simulink model "pedal"  (R2021a)
settings: Solver=FixedStepDiscrete  StartTime=0.0  StopTime=12  FixedStep=1e-3  RelTol=1e-3  EnableMultiTasking=on
undefined symbols (not defined in the file): APP_Modes, sigbuilder_block
settings Model: SILPILModeSetting=veronly  ExtModeTrigDuration=2  Creator=Beshary  LastModifiedBy=Beshary
settings DataIOCC: ExternalInput=[t, S1,S2]  LoadExternalInput=on  SaveFormat=Array
settings OptimizationCC: EnhancedBackFolding=on  PassReuseOutputArgsAs=Individual arguments  ZeroExternalMemoryAtStartup=off  ZeroInternalMemoryAtStartup=off  MaxStackSize=64  OptimizeBlockOrder=speed  DifferentSizesBufferReuse=on  OptimizationCustomize=off  EfficientTunableParamExpr=on
settings DebuggingCC: ParameterTunabilityLossMsg=error
settings HardwareCC: ProdBitPerInt=16  ProdBitPerPointer=16  ProdBitPerSizeT=16  ProdBitPerPtrDiffT=16  ProdLargestAtomicFloat=None  ProdWordSize=8  ProdHWDeviceType=Atmel->AVR
settings SFSimCC: MATLABDynamicMemAlloc=off
settings RTWCC: SystemTargetFile=ert.tlc  HardwareBoard=Arduino Uno  TemplateMakefile=ert_default_tmf  Toolchain=Arduino AVR  BuildConfiguration=Faster Runs
settings CodeAppCC: ForceParamTrailComments=on  IgnoreCustomStorageClasses=off  OperatorAnnotations=on  SimulinkDataObjDesc=on  SFDataObjDesc=on  InsertBlockDesc=on
settings ERTTargetCC: SupportContinuousTime=on  SupportVariableSizeSignals=on  ExtModeStaticAllocSize=250

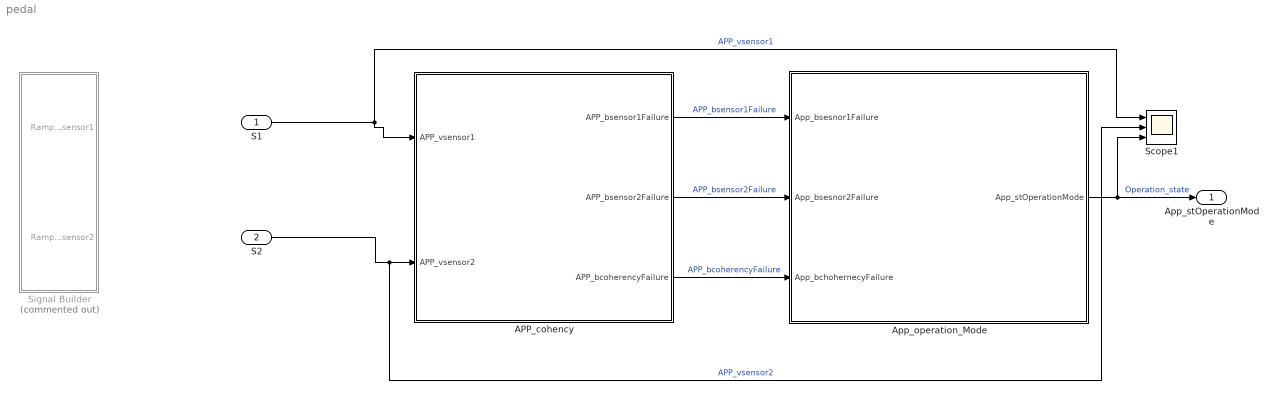
== system pedal ==
  S1 : Inport
  S2 : Inport  Port=2
  APP_cohency : Subsystem
  App_operation_Mode : Subsystem
      mask DialogControl DescGroupVar Prompt: block
  Scope1 : Scope  NumInputPorts=3
  Signal Builder : Subsystem  Tag=STV Subsys  Commented=on  LoadFcn=sigbuilder_block('load');  StartFcn=sigbuilder_block('start');  StopFcn=sigbuilder_block('stop');  ClipboardFcn=sigbuilder_block('clipboard');  mask(Sigbuilder block){tuvar=[0:10]}
      mask help: Simulink:masks:SigbuilderBlock_MD
      mask init:
      | if ~strcmp(get_param(bdroot(gcbh),'SimulationStatus'),'stopped') tuvar = sigbuilder_block('maskInit'); end
      settings: CopyFcn=sigbuilder_block('copy');  DeleteFcn=sigbuilder_block('delete');  ModelCloseFcn=sigbuilder_block('modelClose');  PreSaveFcn=sigbuilder_block('preSave');  PauseFcn=sigbuilder_block('pause');  ContinueFcn=sigbuilder_block('continue');  NameChangeFcn=sigbuilder_block('namechange');  OpenFcn=sigbuilder_block('open',[437.6 199.2 550.4 400 ]);  CloseFcn=sigbuilder_block('close');
      mask Display: plot(0, 0, 100, 100,[2, 2, 32, 32, 2], [68, 8, 8, 68, 68],[32, 2], [38, 38], [32, 19, 2],[53, 60, 44], [32, 17, 17, 2],[16, 16, 31, 31]);txt = getActiveGroup(gcbh);text(2, 100, txt,'verticalAlignment', 'top');
  App_stOperationMode : Outport
  wires:
  App_operation_Mode/1(App_stOperationMode) -> Scope1/3, App_stOperationMode/1  "Operation_state"
  APP_cohency/1(APP_bsensor1Failure) -> App_operation_Mode/1(App_bsesnor1Failure)  "APP_bsensor1Failure"
  APP_cohency/2(APP_bsensor2Failure) -> App_operation_Mode/2(App_bsesnor2Failure)  "APP_bsensor2Failure"
  APP_cohency/3(APP_bcoherencyFailure) -> App_operation_Mode/3(App_bchohernecyFailure)  "APP_bcoherencyFailure"
  S1/1 -> APP_cohency/1(APP_vsensor1), Scope1/1  "APP_vsensor1"
  S2/1 -> Scope1/2, APP_cohency/2(APP_vsensor2)  "APP_vsensor2"

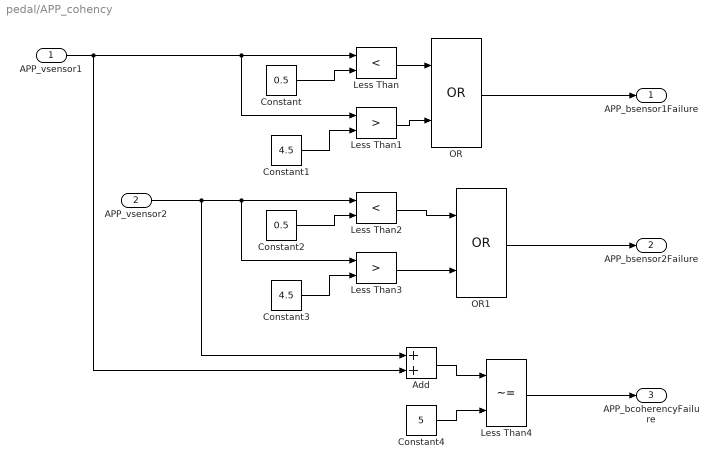
== system pedal/APP_cohency ==
  APP_vsensor1 : Inport
  APP_vsensor2 : Inport  Port=2
  Add : Sum
  Constant : Constant  Value=0.5
  Constant1 : Constant  Value=4.5
  Constant2 : Constant  Value=0.5
  Constant3 : Constant  Value=4.5
  Constant4 : Constant  Value=5
  Less Than : RelationalOperator  Operator=<  OutDataTypeStr=boolean  RndMeth=Simplest
  Less Than1 : RelationalOperator  Operator=>  OutDataTypeStr=boolean  RndMeth=Simplest
  Less Than2 : RelationalOperator  Operator=<  OutDataTypeStr=boolean  RndMeth=Simplest
  Less Than3 : RelationalOperator  Operator=>  OutDataTypeStr=boolean  RndMeth=Simplest
  Less Than4 : RelationalOperator  Operator=~=  OutDataTypeStr=boolean  RndMeth=Simplest
  OR : Logic  Operator=OR  AllPortsSameDT=off  OutDataTypeStr=boolean
  OR1 : Logic  Operator=OR  AllPortsSameDT=off  OutDataTypeStr=boolean
  APP_bsensor1Failure : Outport
  APP_bsensor2Failure : Outport  Port=2
  APP_bcoherencyFailure : Outport  Port=3
  wires:
  APP_vsensor1/1 -> Add/2, Less Than1/1, Less Than/1
  Constant/1 -> Less Than/2
  Less Than/1 -> OR/1
  Constant1/1 -> Less Than1/2
  Less Than1/1 -> OR/2
  OR/1 -> APP_bsensor1Failure/1
  Constant3/1 -> Less Than3/2
  Constant2/1 -> Less Than2/2
  APP_vsensor2/1 -> Add/1, Less Than3/1, Less Than2/1
  Less Than2/1 -> OR1/1
  Less Than3/1 -> OR1/2
  OR1/1 -> APP_bsensor2Failure/1
  Add/1 -> Less Than4/1
  Constant4/1 -> Less Than4/2
  Less Than4/1 -> APP_bcoherencyFailure/1

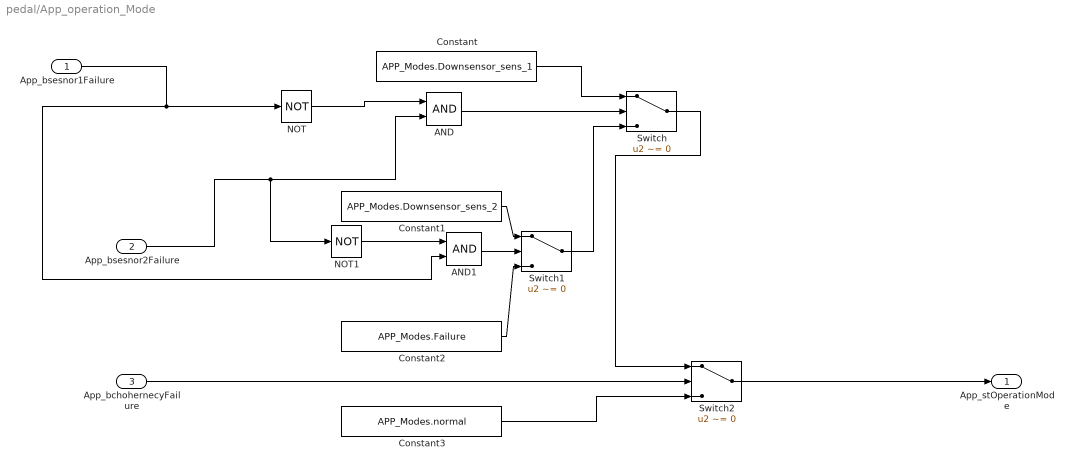
== system pedal/App_operation_Mode ==
  App_bsesnor1Failure : Inport
  App_bsesnor2Failure : Inport  Port=2
  App_bchohernecyFailure : Inport  Port=3
  AND : Logic  AllPortsSameDT=off  OutDataTypeStr=boolean
  AND1 : Logic  AllPortsSameDT=off  OutDataTypeStr=boolean
  Constant : Constant  Value=APP_Modes.Downsensor_sens_1
  Constant1 : Constant  Value=APP_Modes.Downsensor_sens_2
  Constant2 : Constant  Value=APP_Modes.Failure
  Constant3 : Constant  Value=APP_Modes.normal
  NOT : Logic  Operator=NOT  AllPortsSameDT=off  OutDataTypeStr=boolean
  NOT1 : Logic  Operator=NOT  AllPortsSameDT=off  OutDataTypeStr=boolean
  Switch : Switch  Criteria=u2 ~= 0
  Switch1 : Switch  Criteria=u2 ~= 0
  Switch2 : Switch  Criteria=u2 ~= 0
  App_stOperationMode : Outport  OutDataTypeStr=Enum: APP_Modes
  wires:
  NOT/1 -> AND/1
  App_bsesnor1Failure/1 -> NOT/1, AND1/2
  App_bsesnor2Failure/1 -> NOT1/1, AND/2
  AND/1 -> Switch/2
  Constant/1 -> Switch/1
  NOT1/1 -> AND1/1
  AND1/1 -> Switch1/2
  Constant1/1 -> Switch1/1
  Constant2/1 -> Switch1/3
  App_bchohernecyFailure/1 -> Switch2/2
  Switch/1 -> Switch2/1
  Constant3/1 -> Switch2/3
  Switch2/1 -> App_stOperationMode/1
  Switch1/1 -> Switch/3

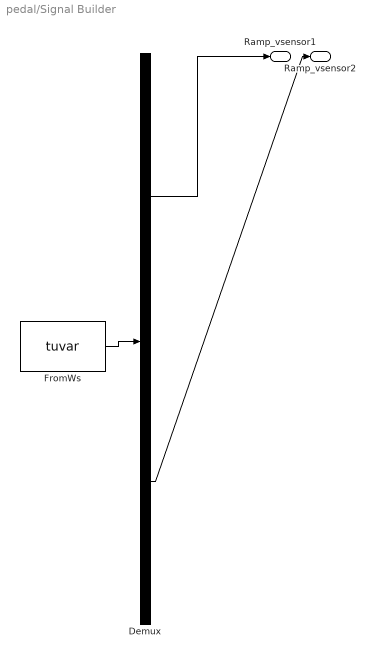
== system pedal/Signal Builder ==
  Demux : Demux  Tag=STV Demux  Outputs=2
      settings: DisplayOption=none
  FromWs : FromWorkspace  Tag=STV FromWs  VariableName=tuvar
      SigBuilderData=|
      | common.afterFinalStr = 'Extrapolate'
      | common.sampleTime = 0
      | dataSet.timeRange = [0 13]
      | dataSet.name = 'Sheet1'
      | sbobj.Name = 'Signal Builder'
      | sbobj.Groups.Name = 'Sheet1'
      | sbobj.Groups.Signals(1).Name = 'Ramp_vsensor1'
      | sbobj.Groups.Signals(1).XData = [0 3 3 5 5 7 7 9 11 11 13]
      | sbobj.Groups.Signals(1).YData = [4.6 4.6 4.5 4.5 0.5 0.5 0.4 0.4 0.4 3 3]
      | sbobj.Groups.Signals(2).Name = 'Ramp_vsensor2'
      | sbobj.Groups.Signals(2).XData = [0 3 3 5 5 7 7 9 9 11 11 13]
      | sbobj.Groups.Signals(2).YData = [4.6 4.6 4.5 4.5 4.6 4.6 0.4 0.4 4.6 4.6 0.4 0.4]
      | sbobj.Groups.TimeRange = [0 13]
  Ramp_vsensor1 : Outport  Tag=STV Outport
  Ramp_vsensor2 : Outport  Tag=STV Outport  Port=2
  wires:
  Demux/1 -> Ramp_vsensor1/1
  FromWs/1 -> Demux/1
  Demux/2 -> Ramp_vsensor2/1
